simulink model "test_bu01_2018b_tuning"  (R2018b)
settings: Solver=FixedStepAuto  StartTime=0.0  StopTime=10  FixedStep=0.001  RelTol=1e-3
model workspace (MAT data in the model file):
  B1 = 0.0229925610147
  B2 = -0.371283802987
  B3 = -0.920624315565
  B4 = -0.0418343375444
  B5 = -0.493210333206
  B6 = 0
  B7 = -0.0892006103314
  B8 = -0.433620647544
  Ixx = 0.8
  Iyy = 2.075
  Izz = 1.25
  K = 0.92
  K1 = 0.96
  M1 = [1 1 -1 0.151123095698]
  M2 = [1 0 1 0.728919165533]
  M3 = [-1 0 -1 0]
  M4 = [-1 1 1 0.279370204784]
  M5 = [0 -1 0 0.953177368176]
  M6 = [0 -1 0 -1]
  M7 = [0 -1 0 0.164756597211]
  M8 = [0 -1 0 0.72330475505]
  Mass = 11.5
  b = 0
libraries: simulink x4, vrlib x4, shared6dof x1
(part 3 of 3)

== system test_bu01_2018b_tuning/Plant/bu01_model/动力系统模型/Motor4_TM_N/TM1654N /螺旋桨模型/螺旋桨气动/计算螺旋桨气动系数 ==
  In1 : Inport
  Bus Selector : BusSelector  OutputSignals=Miu,Lumda
  Mux : Mux  Inputs=6
  计算Cmx : Subsystem
  计算Cmy : Subsystem
  计算Cmz : Subsystem
  计算Ctx : Subsystem
  计算Cty : Subsystem
  计算Ctz : Subsystem
  Out1 : Outport
  wires:
  In1/1 -> Bus Selector/1
  Bus Selector/1 -> 计算Cmz/1(Miu), 计算Cmy/1(Miu), 计算Cmx/1(Miu), 计算Ctz/1(Miu), 计算Cty/1(Miu), 计算Ctx/1(Miu)  "<Miu>"
  Bus Selector/2 -> 计算Cmz/2(Lumda), 计算Cmy/2(Lumda), 计算Cmx/2(Lumda), 计算Ctz/2(Lumda), 计算Ctx/2(Lumda), 计算Cty/2(Lumda)  "<Lumda>"
  计算Ctx/1(Ctx) -> Mux/1  "Ctx"
  计算Cty/1(Cty) -> Mux/2  "Cty"
  计算Ctz/1(Ctz) -> Mux/3  "Ctz"
  计算Cmx/1(Cmx) -> Mux/4  "Cmx"
  计算Cmy/1(Cmy) -> Mux/5  "Cmy"
  计算Cmz/1(Cmz) -> Mux/6  "Cmz"
  Mux/1 -> Out1/1

== system test_bu01_2018b_tuning/Plant/bu01_model/动力系统模型/Motor5_PF_N/PF70mmDuctFanN/涵道风扇模型 /求解涵道风扇气动载荷/Fxp ==
  Vha : Inport
  Vva1 : Inport  Port=2
  Ns : Inport  Port=3
  -0.00000028262 : Gain  Gain=-0.00000028262
  -0.0038 : Gain  Gain=-0.0038
  -0.005 : Gain  Gain=-0.005
  -0.1371 : Gain  Gain=-0.1371
  0.00019569 : Gain  Gain=0.00019569
  Ns^2 : Math  Operator=square  SaturateOnIntegerOverflow=on
  Plus : Sum  Inputs=+++++
  Vha*Ns^2 : Product
  Vha*Vva1 : Product
  Vha*Vva1^2 : Product
  Vha^2 : Math  Operator=square  SaturateOnIntegerOverflow=on
  Vva1^2 : Math  Operator=square  SaturateOnIntegerOverflow=on
  Out1 : Outport
  wires:
  Vha/1 -> Vha*Vva1^2/2, -0.1371/1, Vha^2/1, Vha*Ns^2/1, Vha*Vva1/1  "Vha"
  Vva1/1 -> Vva1^2/1, Vha*Vva1/2  "Vva1"
  Vha*Vva1/1 -> -0.0038/1
  -0.0038/1 -> Plus/1
  Ns/1 -> Ns^2/1  "Ns"
  Vva1^2/1 -> Vha*Vva1^2/1
  Vha*Vva1^2/1 -> 0.00019569/1
  0.00019569/1 -> Plus/2
  -0.1371/1 -> Plus/3
  Vha^2/1 -> -0.005/1
  -0.005/1 -> Plus/4
  Ns^2/1 -> Vha*Ns^2/2
  Vha*Ns^2/1 -> -0.00000028262/1
  -0.00000028262/1 -> Plus/5
  Plus/1 -> Out1/1  "Fxp"

== system test_bu01_2018b_tuning/Plant/bu01_model/动力系统模型/Motor5_PF_N/PF70mmDuctFanN/涵道风扇模型 /求解涵道风扇气动载荷/Fzp ==
  Vha : Inport
  Vva1 : Inport  Port=2
  Ns : Inport  Port=3
  -0.3033 : Gain  Gain=-0.3033
  0.000030466 : Gain  Gain=0.000030466
  0.0019 : Gain  Gain=0.0019
  0.0043 : Gain  Gain=0.0043
  Ns^2 : Math  Operator=square  SaturateOnIntegerOverflow=on
  Plus : Sum  Inputs=++++
  Vha^2 : Math  Operator=square  SaturateOnIntegerOverflow=on
  Vva1^2 : Math  Operator=square  SaturateOnIntegerOverflow=on
  Out1 : Outport
  wires:
  Vha/1 -> Vha^2/1  "Vha"
  Vva1/1 -> -0.3033/1, Vva1^2/1  "Vva1"
  Ns/1 -> Ns^2/1  "Ns"
  -0.3033/1 -> Plus/1
  Vva1^2/1 -> 0.0019/1
  0.0019/1 -> Plus/2
  Vha^2/1 -> 0.0043/1
  0.0043/1 -> Plus/3
  Ns^2/1 -> 0.000030466/1
  0.000030466/1 -> Plus/4
  Plus/1 -> Out1/1  "Fzp"

== system test_bu01_2018b_tuning/Plant/bu01_model/动力系统模型/Motor5_PF_N/PF70mmDuctFanN/涵道风扇模型 /求解涵道风扇气动载荷/Myp ==
  Vha : Inport
  Vva : Inport  Port=2
  Ns : Inport  Port=3
  -0.000000034015 : Gain  Gain=-0.000000034015
  -0.0000031711 : Gain  Gain=-0.0000031711
  -0.0158 : Gain  Gain=-0.0158
  0.000063804 : Gain  Gain=0.000063804
  0.00011649 : Gain  Gain=0.00011649
  Ns^2 : Math  Operator=square  SaturateOnIntegerOverflow=on
  Plus : Sum  Inputs=+++++
  Vha*Ns^2 : Product
  Vha*Vva1 : Product
  Vha*Vva1^2 : Product
  Vha^2 : Math  Operator=square  SaturateOnIntegerOverflow=on
  Vva1^2 : Math  Operator=square  SaturateOnIntegerOverflow=on
  Out1 : Outport
  wires:
  Vha/1 -> Vha*Vva1^2/1, -0.0158/1, Vha^2/1, Vha*Ns^2/1, Vha*Vva1/1  "Vha"
  Vva/1 -> Vha*Vva1/2, Vva1^2/1  "Vva1"
  Ns/1 -> Ns^2/1  "Ns"
  Plus/1 -> Out1/1  "Myp"
  Vha*Vva1/1 -> 0.00011649/1
  0.00011649/1 -> Plus/1
  Vha*Vva1^2/1 -> -0.0000031711/1
  -0.0000031711/1 -> Plus/2
  Vva1^2/1 -> Vha*Vva1^2/2
  -0.0158/1 -> Plus/3
  Vha^2/1 -> 0.000063804/1
  0.000063804/1 -> Plus/4
  -0.000000034015/1 -> Plus/5
  Vha*Ns^2/1 -> -0.000000034015/1
  Ns^2/1 -> Vha*Ns^2/2

== system test_bu01_2018b_tuning/Plant/bu01_model/动力系统模型/Motor5_PF_N/PF70mmDuctFanN/涵道风扇模型 /求解涵道风扇气动载荷/Mzp ==
  Vha : Inport
  Vva1 : Inport  Port=2
  Ns : Inport  Port=3
  -0.0000028793 : Gain  Gain=-0.0000028793
  -0.0002934 : Gain  Gain=-0.0002934
  -0.00035119 : Gain  Gain=-0.00035119
  "0.0000003498 " : Gain  Gain=0.0000003498
  0.000020926 : Gain  Gain=0.000020926
  Ns^2 : Math  Operator=square  SaturateOnIntegerOverflow=on
  Plus : Sum  Inputs=+++++
  Vha^2 : Math  Operator=square  SaturateOnIntegerOverflow=on
  Vva1^2 : Math  Operator=square  SaturateOnIntegerOverflow=on
  Out1 : Outport
  wires:
  Plus/1 -> Out1/1  "Mzp"
  Vha/1 -> Vha^2/1, -0.0002934/1  "Vha"
  Vva1/1 -> Vva1^2/1, -0.00035119/1  "Vva1"
  Ns/1 -> Ns^2/1  "Ns"
  -0.00035119/1 -> Plus/1
  -0.0000028793/1 -> Plus/2
  Vva1^2/1 -> -0.0000028793/1
  -0.0002934/1 -> Plus/3
  0.000020926/1 -> Plus/4
  Vha^2/1 -> 0.000020926/1
  "0.0000003498 "/1 -> Plus/5
  Ns^2/1 -> "0.0000003498 "/1

== system test_bu01_2018b_tuning/Plant/bu01_model/动力系统模型/Motor5_PF_N/PF70mmDuctFanN/涵道风扇模型 /求解涵道风扇气动载荷/切向速度低 ==
  Ax : Inport
  Fp : Inport  Port=2
  Mp : Inport  Port=3
  Bus Creator : BusCreator  Inputs=2
  Matrix Multiply : Product
  Matrix Multiply1 : Product
  Out1 : Outport
  wires:
  Ax/1 -> Matrix Multiply1/2, Matrix Multiply/2  "Ax"
  Fp/1 -> Matrix Multiply/1  "Fp"
  Mp/1 -> Matrix Multiply1/1  "Mp"
  Bus Creator/1 -> Out1/1
  Matrix Multiply/1 -> Bus Creator/1  "Fb"
  Matrix Multiply1/1 -> Bus Creator/2  "Mb"

== system test_bu01_2018b_tuning/Plant/bu01_model/动力系统模型/Motor5_PF_N/PF70mmDuctFanN/涵道风扇模型 /求解涵道风扇气动载荷/需要坐标转换 ==
  Az : Inport
  "[Uba, Vba, Wba]" : Inport  Port=2
  Vva : Inport  Port=3
  Vha : Inport  Port=4
  Fp : Inport  Port=5
  Mp : Inport  Port=6
  Az*Vva : Product
  Az*Vva-Vb : Sum  Inputs=+-
  Bus Creator2 : BusCreator  Inputs=2
  Cross Product : vrlib/Utilities/Cross Product
      settings: SourceProductBaseCode=VR
  Divide : Product  Inputs=*/
  Fxb : DotProduct  InputSameDT=on  OutDataTypeStr=Inherit: Inherit via internal rule
  Fyb : DotProduct  InputSameDT=on  OutDataTypeStr=Inherit: Inherit via internal rule
  Fzb : DotProduct  InputSameDT=on  OutDataTypeStr=Inherit: Inherit via internal rule
  Mux : Mux  Inputs=3
  Mux1 : Mux  Inputs=3
  Mxb : DotProduct  InputSameDT=on  OutDataTypeStr=Inherit: Inherit via internal rule
  Myb : DotProduct  InputSameDT=on  OutDataTypeStr=Inherit: Inherit via internal rule
  Mzb : DotProduct  InputSameDT=on  OutDataTypeStr=Inherit: Inherit via internal rule
  Saturation : Saturate  UpperLimit=inf  LowerLimit=eps
  Out1 : Outport
  wires:
  Vva/1 -> Az*Vva/2  "Vva"
  Az/1 -> Cross Product/1, Fzb/2, Mzb/2, Az*Vva/1  "Azb"
  Az*Vva/1 -> Az*Vva-Vb/1
  "[Uba, Vba, Wba]"/1 -> Az*Vva-Vb/2  "Vb"
  Az*Vva-Vb/1 -> Divide/1
  Divide/1 -> Cross Product/2, Mxb/2, Fxb/2  "Axb"
  Cross Product/1 -> Myb/2, Fyb/2  "Ayb"
  Fp/1 -> Fzb/1, Fyb/1, Fxb/1
  Mp/1 -> Mzb/1, Myb/1, Mxb/1
  Fxb/1 -> Mux1/1  "Fxb"
  Fyb/1 -> Mux1/2  "Fyb"
  Fzb/1 -> Mux1/3  "Fzb"
  Mxb/1 -> Mux/1  "Mxb"
  Myb/1 -> Mux/2  "Myb"
  Mzb/1 -> Mux/3  "Mzb"
  Mux1/1 -> Bus Creator2/1  "Fb"
  Mux/1 -> Bus Creator2/2  "Mb"
  Bus Creator2/1 -> Out1/1
  Vha/1 -> Saturation/1  "Vha"
  Saturation/1 -> Divide/2

== system test_bu01_2018b_tuning/Plant/bu01_model/动力系统模型/Motor6_PF_N/PF70mmDuctFanN/涵道风扇模型 /求解涵道风扇气动载荷/Fxp ==
  Vha : Inport
  Vva1 : Inport  Port=2
  Ns : Inport  Port=3
  -0.00000028262 : Gain  Gain=-0.00000028262
  -0.0038 : Gain  Gain=-0.0038
  -0.005 : Gain  Gain=-0.005
  -0.1371 : Gain  Gain=-0.1371
  0.00019569 : Gain  Gain=0.00019569
  Ns^2 : Math  Operator=square  SaturateOnIntegerOverflow=on
  Plus : Sum  Inputs=+++++
  Vha*Ns^2 : Product
  Vha*Vva1 : Product
  Vha*Vva1^2 : Product
  Vha^2 : Math  Operator=square  SaturateOnIntegerOverflow=on
  Vva1^2 : Math  Operator=square  SaturateOnIntegerOverflow=on
  Out1 : Outport
  wires:
  Vha/1 -> Vha*Vva1^2/2, -0.1371/1, Vha^2/1, Vha*Ns^2/1, Vha*Vva1/1  "Vha"
  Vva1/1 -> Vva1^2/1, Vha*Vva1/2  "Vva1"
  Vha*Vva1/1 -> -0.0038/1
  -0.0038/1 -> Plus/1
  Ns/1 -> Ns^2/1  "Ns"
  Vva1^2/1 -> Vha*Vva1^2/1
  Vha*Vva1^2/1 -> 0.00019569/1
  0.00019569/1 -> Plus/2
  -0.1371/1 -> Plus/3
  Vha^2/1 -> -0.005/1
  -0.005/1 -> Plus/4
  Ns^2/1 -> Vha*Ns^2/2
  Vha*Ns^2/1 -> -0.00000028262/1
  -0.00000028262/1 -> Plus/5
  Plus/1 -> Out1/1  "Fxp"

== system test_bu01_2018b_tuning/Plant/bu01_model/动力系统模型/Motor6_PF_N/PF70mmDuctFanN/涵道风扇模型 /求解涵道风扇气动载荷/Fzp ==
  Vha : Inport
  Vva1 : Inport  Port=2
  Ns : Inport  Port=3
  -0.3033 : Gain  Gain=-0.3033
  0.000030466 : Gain  Gain=0.000030466
  0.0019 : Gain  Gain=0.0019
  0.0043 : Gain  Gain=0.0043
  Ns^2 : Math  Operator=square  SaturateOnIntegerOverflow=on
  Plus : Sum  Inputs=++++
  Vha^2 : Math  Operator=square  SaturateOnIntegerOverflow=on
  Vva1^2 : Math  Operator=square  SaturateOnIntegerOverflow=on
  Out1 : Outport
  wires:
  Vha/1 -> Vha^2/1  "Vha"
  Vva1/1 -> -0.3033/1, Vva1^2/1  "Vva1"
  Ns/1 -> Ns^2/1  "Ns"
  -0.3033/1 -> Plus/1
  Vva1^2/1 -> 0.0019/1
  0.0019/1 -> Plus/2
  Vha^2/1 -> 0.0043/1
  0.0043/1 -> Plus/3
  Ns^2/1 -> 0.000030466/1
  0.000030466/1 -> Plus/4
  Plus/1 -> Out1/1  "Fzp"

== system test_bu01_2018b_tuning/Plant/bu01_model/动力系统模型/Motor6_PF_N/PF70mmDuctFanN/涵道风扇模型 /求解涵道风扇气动载荷/Myp ==
  Vha : Inport
  Vva : Inport  Port=2
  Ns : Inport  Port=3
  -0.000000034015 : Gain  Gain=-0.000000034015
  -0.0000031711 : Gain  Gain=-0.0000031711
  -0.0158 : Gain  Gain=-0.0158
  0.000063804 : Gain  Gain=0.000063804
  0.00011649 : Gain  Gain=0.00011649
  Ns^2 : Math  Operator=square  SaturateOnIntegerOverflow=on
  Plus : Sum  Inputs=+++++
  Vha*Ns^2 : Product
  Vha*Vva1 : Product
  Vha*Vva1^2 : Product
  Vha^2 : Math  Operator=square  SaturateOnIntegerOverflow=on
  Vva1^2 : Math  Operator=square  SaturateOnIntegerOverflow=on
  Out1 : Outport
  wires:
  Vha/1 -> Vha*Vva1^2/1, -0.0158/1, Vha^2/1, Vha*Ns^2/1, Vha*Vva1/1  "Vha"
  Vva/1 -> Vha*Vva1/2, Vva1^2/1  "Vva1"
  Ns/1 -> Ns^2/1  "Ns"
  Plus/1 -> Out1/1  "Myp"
  Vha*Vva1/1 -> 0.00011649/1
  0.00011649/1 -> Plus/1
  Vha*Vva1^2/1 -> -0.0000031711/1
  -0.0000031711/1 -> Plus/2
  Vva1^2/1 -> Vha*Vva1^2/2
  -0.0158/1 -> Plus/3
  Vha^2/1 -> 0.000063804/1
  0.000063804/1 -> Plus/4
  -0.000000034015/1 -> Plus/5
  Vha*Ns^2/1 -> -0.000000034015/1
  Ns^2/1 -> Vha*Ns^2/2

== system test_bu01_2018b_tuning/Plant/bu01_model/动力系统模型/Motor6_PF_N/PF70mmDuctFanN/涵道风扇模型 /求解涵道风扇气动载荷/Mzp ==
  Vha : Inport
  Vva1 : Inport  Port=2
  Ns : Inport  Port=3
  -0.0000028793 : Gain  Gain=-0.0000028793
  -0.0002934 : Gain  Gain=-0.0002934
  -0.00035119 : Gain  Gain=-0.00035119
  "0.0000003498 " : Gain  Gain=0.0000003498
  0.000020926 : Gain  Gain=0.000020926
  Ns^2 : Math  Operator=square  SaturateOnIntegerOverflow=on
  Plus : Sum  Inputs=+++++
  Vha^2 : Math  Operator=square  SaturateOnIntegerOverflow=on
  Vva1^2 : Math  Operator=square  SaturateOnIntegerOverflow=on
  Out1 : Outport
  wires:
  Plus/1 -> Out1/1  "Mzp"
  Vha/1 -> Vha^2/1, -0.0002934/1  "Vha"
  Vva1/1 -> Vva1^2/1, -0.00035119/1  "Vva1"
  Ns/1 -> Ns^2/1  "Ns"
  -0.00035119/1 -> Plus/1
  -0.0000028793/1 -> Plus/2
  Vva1^2/1 -> -0.0000028793/1
  -0.0002934/1 -> Plus/3
  0.000020926/1 -> Plus/4
  Vha^2/1 -> 0.000020926/1
  "0.0000003498 "/1 -> Plus/5
  Ns^2/1 -> "0.0000003498 "/1

== system test_bu01_2018b_tuning/Plant/bu01_model/动力系统模型/Motor6_PF_N/PF70mmDuctFanN/涵道风扇模型 /求解涵道风扇气动载荷/切向速度低 ==
  Ax : Inport
  Fp : Inport  Port=2
  Mp : Inport  Port=3
  Bus Creator : BusCreator  Inputs=2
  Matrix Multiply : Product
  Matrix Multiply1 : Product
  Out1 : Outport
  wires:
  Ax/1 -> Matrix Multiply1/2, Matrix Multiply/2  "Ax"
  Fp/1 -> Matrix Multiply/1  "Fp"
  Mp/1 -> Matrix Multiply1/1  "Mp"
  Bus Creator/1 -> Out1/1
  Matrix Multiply/1 -> Bus Creator/1  "Fb"
  Matrix Multiply1/1 -> Bus Creator/2  "Mb"

== system test_bu01_2018b_tuning/Plant/bu01_model/动力系统模型/Motor6_PF_N/PF70mmDuctFanN/涵道风扇模型 /求解涵道风扇气动载荷/需要坐标转换 ==
  Az : Inport
  "[Uba, Vba, Wba]" : Inport  Port=2
  Vva : Inport  Port=3
  Vha : Inport  Port=4
  Fp : Inport  Port=5
  Mp : Inport  Port=6
  Az*Vva : Product
  Az*Vva-Vb : Sum  Inputs=+-
  Bus Creator2 : BusCreator  Inputs=2
  Cross Product : vrlib/Utilities/Cross Product
      settings: SourceProductBaseCode=VR
  Divide : Product  Inputs=*/
  Fxb : DotProduct  InputSameDT=on  OutDataTypeStr=Inherit: Inherit via internal rule
  Fyb : DotProduct  InputSameDT=on  OutDataTypeStr=Inherit: Inherit via internal rule
  Fzb : DotProduct  InputSameDT=on  OutDataTypeStr=Inherit: Inherit via internal rule
  Mux : Mux  Inputs=3
  Mux1 : Mux  Inputs=3
  Mxb : DotProduct  InputSameDT=on  OutDataTypeStr=Inherit: Inherit via internal rule
  Myb : DotProduct  InputSameDT=on  OutDataTypeStr=Inherit: Inherit via internal rule
  Mzb : DotProduct  InputSameDT=on  OutDataTypeStr=Inherit: Inherit via internal rule
  Saturation : Saturate  UpperLimit=inf  LowerLimit=eps
  Out1 : Outport
  wires:
  Vva/1 -> Az*Vva/2  "Vva"
  Az/1 -> Cross Product/1, Fzb/2, Mzb/2, Az*Vva/1  "Azb"
  Az*Vva/1 -> Az*Vva-Vb/1
  "[Uba, Vba, Wba]"/1 -> Az*Vva-Vb/2  "Vb"
  Az*Vva-Vb/1 -> Divide/1
  Divide/1 -> Cross Product/2, Mxb/2, Fxb/2  "Axb"
  Cross Product/1 -> Myb/2, Fyb/2  "Ayb"
  Fp/1 -> Fzb/1, Fyb/1, Fxb/1
  Mp/1 -> Mzb/1, Myb/1, Mxb/1
  Fxb/1 -> Mux1/1  "Fxb"
  Fyb/1 -> Mux1/2  "Fyb"
  Fzb/1 -> Mux1/3  "Fzb"
  Mxb/1 -> Mux/1  "Mxb"
  Myb/1 -> Mux/2  "Myb"
  Mzb/1 -> Mux/3  "Mzb"
  Mux1/1 -> Bus Creator2/1  "Fb"
  Mux/1 -> Bus Creator2/2  "Mb"
  Bus Creator2/1 -> Out1/1
  Vha/1 -> Saturation/1  "Vha"
  Saturation/1 -> Divide/2

== system test_bu01_2018b_tuning/Plant/bu01_model/动力系统模型/Motor7_PF_N/PF70mmDuctFanN/涵道风扇模型 /求解涵道风扇气动载荷/Fxp ==
  Vha : Inport
  Vva1 : Inport  Port=2
  Ns : Inport  Port=3
  -0.00000028262 : Gain  Gain=-0.00000028262
  -0.0038 : Gain  Gain=-0.0038
  -0.005 : Gain  Gain=-0.005
  -0.1371 : Gain  Gain=-0.1371
  0.00019569 : Gain  Gain=0.00019569
  Ns^2 : Math  Operator=square  SaturateOnIntegerOverflow=on
  Plus : Sum  Inputs=+++++
  Vha*Ns^2 : Product
  Vha*Vva1 : Product
  Vha*Vva1^2 : Product
  Vha^2 : Math  Operator=square  SaturateOnIntegerOverflow=on
  Vva1^2 : Math  Operator=square  SaturateOnIntegerOverflow=on
  Out1 : Outport
  wires:
  Vha/1 -> Vha*Vva1^2/2, -0.1371/1, Vha^2/1, Vha*Ns^2/1, Vha*Vva1/1  "Vha"
  Vva1/1 -> Vva1^2/1, Vha*Vva1/2  "Vva1"
  Vha*Vva1/1 -> -0.0038/1
  -0.0038/1 -> Plus/1
  Ns/1 -> Ns^2/1  "Ns"
  Vva1^2/1 -> Vha*Vva1^2/1
  Vha*Vva1^2/1 -> 0.00019569/1
  0.00019569/1 -> Plus/2
  -0.1371/1 -> Plus/3
  Vha^2/1 -> -0.005/1
  -0.005/1 -> Plus/4
  Ns^2/1 -> Vha*Ns^2/2
  Vha*Ns^2/1 -> -0.00000028262/1
  -0.00000028262/1 -> Plus/5
  Plus/1 -> Out1/1  "Fxp"

== system test_bu01_2018b_tuning/Plant/bu01_model/动力系统模型/Motor7_PF_N/PF70mmDuctFanN/涵道风扇模型 /求解涵道风扇气动载荷/Fzp ==
  Vha : Inport
  Vva1 : Inport  Port=2
  Ns : Inport  Port=3
  -0.3033 : Gain  Gain=-0.3033
  0.000030466 : Gain  Gain=0.000030466
  0.0019 : Gain  Gain=0.0019
  0.0043 : Gain  Gain=0.0043
  Ns^2 : Math  Operator=square  SaturateOnIntegerOverflow=on
  Plus : Sum  Inputs=++++
  Vha^2 : Math  Operator=square  SaturateOnIntegerOverflow=on
  Vva1^2 : Math  Operator=square  SaturateOnIntegerOverflow=on
  Out1 : Outport
  wires:
  Vha/1 -> Vha^2/1  "Vha"
  Vva1/1 -> -0.3033/1, Vva1^2/1  "Vva1"
  Ns/1 -> Ns^2/1  "Ns"
  -0.3033/1 -> Plus/1
  Vva1^2/1 -> 0.0019/1
  0.0019/1 -> Plus/2
  Vha^2/1 -> 0.0043/1
  0.0043/1 -> Plus/3
  Ns^2/1 -> 0.000030466/1
  0.000030466/1 -> Plus/4
  Plus/1 -> Out1/1  "Fzp"

== system test_bu01_2018b_tuning/Plant/bu01_model/动力系统模型/Motor7_PF_N/PF70mmDuctFanN/涵道风扇模型 /求解涵道风扇气动载荷/Myp ==
  Vha : Inport
  Vva : Inport  Port=2
  Ns : Inport  Port=3
  -0.000000034015 : Gain  Gain=-0.000000034015
  -0.0000031711 : Gain  Gain=-0.0000031711
  -0.0158 : Gain  Gain=-0.0158
  0.000063804 : Gain  Gain=0.000063804
  0.00011649 : Gain  Gain=0.00011649
  Ns^2 : Math  Operator=square  SaturateOnIntegerOverflow=on
  Plus : Sum  Inputs=+++++
  Vha*Ns^2 : Product
  Vha*Vva1 : Product
  Vha*Vva1^2 : Product
  Vha^2 : Math  Operator=square  SaturateOnIntegerOverflow=on
  Vva1^2 : Math  Operator=square  SaturateOnIntegerOverflow=on
  Out1 : Outport
  wires:
  Vha/1 -> Vha*Vva1^2/1, -0.0158/1, Vha^2/1, Vha*Ns^2/1, Vha*Vva1/1  "Vha"
  Vva/1 -> Vha*Vva1/2, Vva1^2/1  "Vva1"
  Ns/1 -> Ns^2/1  "Ns"
  Plus/1 -> Out1/1  "Myp"
  Vha*Vva1/1 -> 0.00011649/1
  0.00011649/1 -> Plus/1
  Vha*Vva1^2/1 -> -0.0000031711/1
  -0.0000031711/1 -> Plus/2
  Vva1^2/1 -> Vha*Vva1^2/2
  -0.0158/1 -> Plus/3
  Vha^2/1 -> 0.000063804/1
  0.000063804/1 -> Plus/4
  -0.000000034015/1 -> Plus/5
  Vha*Ns^2/1 -> -0.000000034015/1
  Ns^2/1 -> Vha*Ns^2/2

== system test_bu01_2018b_tuning/Plant/bu01_model/动力系统模型/Motor7_PF_N/PF70mmDuctFanN/涵道风扇模型 /求解涵道风扇气动载荷/Mzp ==
  Vha : Inport
  Vva1 : Inport  Port=2
  Ns : Inport  Port=3
  -0.0000028793 : Gain  Gain=-0.0000028793
  -0.0002934 : Gain  Gain=-0.0002934
  -0.00035119 : Gain  Gain=-0.00035119
  "0.0000003498 " : Gain  Gain=0.0000003498
  0.000020926 : Gain  Gain=0.000020926
  Ns^2 : Math  Operator=square  SaturateOnIntegerOverflow=on
  Plus : Sum  Inputs=+++++
  Vha^2 : Math  Operator=square  SaturateOnIntegerOverflow=on
  Vva1^2 : Math  Operator=square  SaturateOnIntegerOverflow=on
  Out1 : Outport
  wires:
  Plus/1 -> Out1/1  "Mzp"
  Vha/1 -> Vha^2/1, -0.0002934/1  "Vha"
  Vva1/1 -> Vva1^2/1, -0.00035119/1  "Vva1"
  Ns/1 -> Ns^2/1  "Ns"
  -0.00035119/1 -> Plus/1
  -0.0000028793/1 -> Plus/2
  Vva1^2/1 -> -0.0000028793/1
  -0.0002934/1 -> Plus/3
  0.000020926/1 -> Plus/4
  Vha^2/1 -> 0.000020926/1
  "0.0000003498 "/1 -> Plus/5
  Ns^2/1 -> "0.0000003498 "/1

== system test_bu01_2018b_tuning/Plant/bu01_model/动力系统模型/Motor7_PF_N/PF70mmDuctFanN/涵道风扇模型 /求解涵道风扇气动载荷/切向速度低 ==
  Ax : Inport
  Fp : Inport  Port=2
  Mp : Inport  Port=3
  Bus Creator : BusCreator  Inputs=2
  Matrix Multiply : Product
  Matrix Multiply1 : Product
  Out1 : Outport
  wires:
  Ax/1 -> Matrix Multiply1/2, Matrix Multiply/2  "Ax"
  Fp/1 -> Matrix Multiply/1  "Fp"
  Mp/1 -> Matrix Multiply1/1  "Mp"
  Bus Creator/1 -> Out1/1
  Matrix Multiply/1 -> Bus Creator/1  "Fb"
  Matrix Multiply1/1 -> Bus Creator/2  "Mb"

== system test_bu01_2018b_tuning/Plant/bu01_model/动力系统模型/Motor7_PF_N/PF70mmDuctFanN/涵道风扇模型 /求解涵道风扇气动载荷/需要坐标转换 ==
  Az : Inport
  "[Uba, Vba, Wba]" : Inport  Port=2
  Vva : Inport  Port=3
  Vha : Inport  Port=4
  Fp : Inport  Port=5
  Mp : Inport  Port=6
  Az*Vva : Product
  Az*Vva-Vb : Sum  Inputs=+-
  Bus Creator2 : BusCreator  Inputs=2
  Cross Product : vrlib/Utilities/Cross Product
      settings: SourceProductBaseCode=VR
  Divide : Product  Inputs=*/
  Fxb : DotProduct  InputSameDT=on  OutDataTypeStr=Inherit: Inherit via internal rule
  Fyb : DotProduct  InputSameDT=on  OutDataTypeStr=Inherit: Inherit via internal rule
  Fzb : DotProduct  InputSameDT=on  OutDataTypeStr=Inherit: Inherit via internal rule
  Mux : Mux  Inputs=3
  Mux1 : Mux  Inputs=3
  Mxb : DotProduct  InputSameDT=on  OutDataTypeStr=Inherit: Inherit via internal rule
  Myb : DotProduct  InputSameDT=on  OutDataTypeStr=Inherit: Inherit via internal rule
  Mzb : DotProduct  InputSameDT=on  OutDataTypeStr=Inherit: Inherit via internal rule
  Saturation : Saturate  UpperLimit=inf  LowerLimit=eps
  Out1 : Outport
  wires:
  Vva/1 -> Az*Vva/2  "Vva"
  Az/1 -> Cross Product/1, Fzb/2, Mzb/2, Az*Vva/1  "Azb"
  Az*Vva/1 -> Az*Vva-Vb/1
  "[Uba, Vba, Wba]"/1 -> Az*Vva-Vb/2  "Vb"
  Az*Vva-Vb/1 -> Divide/1
  Divide/1 -> Cross Product/2, Mxb/2, Fxb/2  "Axb"
  Cross Product/1 -> Myb/2, Fyb/2  "Ayb"
  Fp/1 -> Fzb/1, Fyb/1, Fxb/1
  Mp/1 -> Mzb/1, Myb/1, Mxb/1
  Fxb/1 -> Mux1/1  "Fxb"
  Fyb/1 -> Mux1/2  "Fyb"
  Fzb/1 -> Mux1/3  "Fzb"
  Mxb/1 -> Mux/1  "Mxb"
  Myb/1 -> Mux/2  "Myb"
  Mzb/1 -> Mux/3  "Mzb"
  Mux1/1 -> Bus Creator2/1  "Fb"
  Mux/1 -> Bus Creator2/2  "Mb"
  Bus Creator2/1 -> Out1/1
  Vha/1 -> Saturation/1  "Vha"
  Saturation/1 -> Divide/2

== system test_bu01_2018b_tuning/Plant/bu01_model/动力系统模型/Motor8_PF_N/PF70mmDuctFanN/涵道风扇模型 /求解涵道风扇气动载荷/Fxp ==
  Vha : Inport
  Vva1 : Inport  Port=2
  Ns : Inport  Port=3
  -0.00000028262 : Gain  Gain=-0.00000028262
  -0.0038 : Gain  Gain=-0.0038
  -0.005 : Gain  Gain=-0.005
  -0.1371 : Gain  Gain=-0.1371
  0.00019569 : Gain  Gain=0.00019569
  Ns^2 : Math  Operator=square  SaturateOnIntegerOverflow=on
  Plus : Sum  Inputs=+++++
  Vha*Ns^2 : Product
  Vha*Vva1 : Product
  Vha*Vva1^2 : Product
  Vha^2 : Math  Operator=square  SaturateOnIntegerOverflow=on
  Vva1^2 : Math  Operator=square  SaturateOnIntegerOverflow=on
  Out1 : Outport
  wires:
  Plus/1 -> Out1/1  "Fxp"
  -0.00000028262/1 -> Plus/5
  Vha*Ns^2/1 -> -0.00000028262/1
  Ns^2/1 -> Vha*Ns^2/2
  -0.005/1 -> Plus/4
  Vha^2/1 -> -0.005/1
  -0.1371/1 -> Plus/3
  0.00019569/1 -> Plus/2
  Vha*Vva1^2/1 -> 0.00019569/1
  Vva1^2/1 -> Vha*Vva1^2/1
  Ns/1 -> Ns^2/1  "Ns"
  -0.0038/1 -> Plus/1
  Vha*Vva1/1 -> -0.0038/1
  Vva1/1 -> Vha*Vva1/2, Vva1^2/1  "Vva1"
  Vha/1 -> Vha*Vva1/1, Vha*Ns^2/1, Vha^2/1, -0.1371/1, Vha*Vva1^2/2  "Vha"

== system test_bu01_2018b_tuning/Plant/bu01_model/动力系统模型/Motor8_PF_N/PF70mmDuctFanN/涵道风扇模型 /求解涵道风扇气动载荷/Fzp ==
  Vha : Inport
  Vva1 : Inport  Port=2
  Ns : Inport  Port=3
  -0.3033 : Gain  Gain=-0.3033
  0.000030466 : Gain  Gain=0.000030466
  0.0019 : Gain  Gain=0.0019
  0.0043 : Gain  Gain=0.0043
  Ns^2 : Math  Operator=square  SaturateOnIntegerOverflow=on
  Plus : Sum  Inputs=++++
  Vha^2 : Math  Operator=square  SaturateOnIntegerOverflow=on
  Vva1^2 : Math  Operator=square  SaturateOnIntegerOverflow=on
  Out1 : Outport
  wires:
  Plus/1 -> Out1/1  "Fzp"
  0.000030466/1 -> Plus/4
  Ns^2/1 -> 0.000030466/1
  0.0043/1 -> Plus/3
  Vha^2/1 -> 0.0043/1
  0.0019/1 -> Plus/2
  Vva1^2/1 -> 0.0019/1
  -0.3033/1 -> Plus/1
  Ns/1 -> Ns^2/1  "Ns"
  Vva1/1 -> Vva1^2/1, -0.3033/1  "Vva1"
  Vha/1 -> Vha^2/1  "Vha"

== system test_bu01_2018b_tuning/Plant/bu01_model/动力系统模型/Motor8_PF_N/PF70mmDuctFanN/涵道风扇模型 /求解涵道风扇气动载荷/Myp ==
  Vha : Inport
  Vva : Inport  Port=2
  Ns : Inport  Port=3
  -0.000000034015 : Gain  Gain=-0.000000034015
  -0.0000031711 : Gain  Gain=-0.0000031711
  -0.0158 : Gain  Gain=-0.0158
  0.000063804 : Gain  Gain=0.000063804
  0.00011649 : Gain  Gain=0.00011649
  Ns^2 : Math  Operator=square  SaturateOnIntegerOverflow=on
  Plus : Sum  Inputs=+++++
  Vha*Ns^2 : Product
  Vha*Vva1 : Product
  Vha*Vva1^2 : Product
  Vha^2 : Math  Operator=square  SaturateOnIntegerOverflow=on
  Vva1^2 : Math  Operator=square  SaturateOnIntegerOverflow=on
  Out1 : Outport
  wires:
  Ns^2/1 -> Vha*Ns^2/2
  Vha*Ns^2/1 -> -0.000000034015/1
  -0.000000034015/1 -> Plus/5
  0.000063804/1 -> Plus/4
  Vha^2/1 -> 0.000063804/1
  -0.0158/1 -> Plus/3
  Vva1^2/1 -> Vha*Vva1^2/2
  -0.0000031711/1 -> Plus/2
  Vha*Vva1^2/1 -> -0.0000031711/1
  0.00011649/1 -> Plus/1
  Vha*Vva1/1 -> 0.00011649/1
  Plus/1 -> Out1/1  "Myp"
  Ns/1 -> Ns^2/1  "Ns"
  Vva/1 -> Vva1^2/1, Vha*Vva1/2  "Vva1"
  Vha/1 -> Vha*Vva1/1, Vha*Ns^2/1, Vha^2/1, -0.0158/1, Vha*Vva1^2/1  "Vha"

== system test_bu01_2018b_tuning/Plant/bu01_model/动力系统模型/Motor8_PF_N/PF70mmDuctFanN/涵道风扇模型 /求解涵道风扇气动载荷/Mzp ==
  Vha : Inport
  Vva1 : Inport  Port=2
  Ns : Inport  Port=3
  -0.0000028793 : Gain  Gain=-0.0000028793
  -0.0002934 : Gain  Gain=-0.0002934
  -0.00035119 : Gain  Gain=-0.00035119
  "0.0000003498 " : Gain  Gain=0.0000003498
  0.000020926 : Gain  Gain=0.000020926
  Ns^2 : Math  Operator=square  SaturateOnIntegerOverflow=on
  Plus : Sum  Inputs=+++++
  Vha^2 : Math  Operator=square  SaturateOnIntegerOverflow=on
  Vva1^2 : Math  Operator=square  SaturateOnIntegerOverflow=on
  Out1 : Outport
  wires:
  Ns^2/1 -> "0.0000003498 "/1
  "0.0000003498 "/1 -> Plus/5
  Vha^2/1 -> 0.000020926/1
  0.000020926/1 -> Plus/4
  -0.0002934/1 -> Plus/3
  Vva1^2/1 -> -0.0000028793/1
  -0.0000028793/1 -> Plus/2
  -0.00035119/1 -> Plus/1
  Ns/1 -> Ns^2/1  "Ns"
  Vva1/1 -> -0.00035119/1, Vva1^2/1  "Vva1"
  Vha/1 -> -0.0002934/1, Vha^2/1  "Vha"
  Plus/1 -> Out1/1  "Mzp"

== system test_bu01_2018b_tuning/Plant/bu01_model/动力系统模型/Motor8_PF_N/PF70mmDuctFanN/涵道风扇模型 /求解涵道风扇气动载荷/切向速度低 ==
  Ax : Inport
  Fp : Inport  Port=2
  Mp : Inport  Port=3
  Bus Creator : BusCreator  Inputs=2
  Matrix Multiply : Product
  Matrix Multiply1 : Product
  Out1 : Outport
  wires:
  Matrix Multiply1/1 -> Bus Creator/2  "Mb"
  Matrix Multiply/1 -> Bus Creator/1  "Fb"
  Bus Creator/1 -> Out1/1
  Mp/1 -> Matrix Multiply1/1  "Mp"
  Fp/1 -> Matrix Multiply/1  "Fp"
  Ax/1 -> Matrix Multiply/2, Matrix Multiply1/2  "Ax"

== system test_bu01_2018b_tuning/Plant/bu01_model/动力系统模型/Motor8_PF_N/PF70mmDuctFanN/涵道风扇模型 /求解涵道风扇气动载荷/需要坐标转换 ==
  Az : Inport
  "[Uba, Vba, Wba]" : Inport  Port=2
  Vva : Inport  Port=3
  Vha : Inport  Port=4
  Fp : Inport  Port=5
  Mp : Inport  Port=6
  Az*Vva : Product
  Az*Vva-Vb : Sum  Inputs=+-
  Bus Creator2 : BusCreator  Inputs=2
  Cross Product : vrlib/Utilities/Cross Product
      settings: SourceProductBaseCode=VR
  Divide : Product  Inputs=*/
  Fxb : DotProduct  InputSameDT=on  OutDataTypeStr=Inherit: Inherit via internal rule
  Fyb : DotProduct  InputSameDT=on  OutDataTypeStr=Inherit: Inherit via internal rule
  Fzb : DotProduct  InputSameDT=on  OutDataTypeStr=Inherit: Inherit via internal rule
  Mux : Mux  Inputs=3
  Mux1 : Mux  Inputs=3
  Mxb : DotProduct  InputSameDT=on  OutDataTypeStr=Inherit: Inherit via internal rule
  Myb : DotProduct  InputSameDT=on  OutDataTypeStr=Inherit: Inherit via internal rule
  Mzb : DotProduct  InputSameDT=on  OutDataTypeStr=Inherit: Inherit via internal rule
  Saturation : Saturate  UpperLimit=inf  LowerLimit=eps
  Out1 : Outport
  wires:
  Bus Creator2/1 -> Out1/1
  Mux/1 -> Bus Creator2/2  "Mb"
  Mux1/1 -> Bus Creator2/1  "Fb"
  Mzb/1 -> Mux/3  "Mzb"
  Myb/1 -> Mux/2  "Myb"
  Mxb/1 -> Mux/1  "Mxb"
  Fzb/1 -> Mux1/3  "Fzb"
  Fyb/1 -> Mux1/2  "Fyb"
  Fxb/1 -> Mux1/1  "Fxb"
  Mp/1 -> Mxb/1, Myb/1, Mzb/1
  Fp/1 -> Fxb/1, Fyb/1, Fzb/1
  Cross Product/1 -> Fyb/2, Myb/2  "Ayb"
  Divide/1 -> Fxb/2, Mxb/2, Cross Product/2  "Axb"
  Az*Vva-Vb/1 -> Divide/1
  "[Uba, Vba, Wba]"/1 -> Az*Vva-Vb/2  "Vb"
  Az*Vva/1 -> Az*Vva-Vb/1
  Az/1 -> Az*Vva/1, Mzb/2, Fzb/2, Cross Product/1  "Azb"
  Vva/1 -> Az*Vva/2  "Vva"
  Vha/1 -> Saturation/1  "Vha"
  Saturation/1 -> Divide/2

== system test_bu01_2018b_tuning/Plant/bu01_model/动力系统模型/Motor1_TM_P/TM1654P /螺旋桨模型/螺旋桨气动/计算螺旋桨气动系数/计算Cmx ==
  Miu : Inport
  Lumda : Inport  Port=2
  Add : Sum  Inputs=++--
  Constant : Constant  Value=0.0101
  Gain : Gain  Gain=0.0041
  Gain1 : Gain  Gain=0.009
  Gain2 : Gain  Gain=0.0032
  Multiply : Product
  Square : Math  Operator=square  SaturateOnIntegerOverflow=on
  Cmx : Outport
  wires:
  Multiply/1 -> Cmx/1  "Cmx"
  Lumda/1 -> Square/1, Gain1/1
  Gain2/1 -> Add/4
  Square/1 -> Gain2/1
  Gain/1 -> Add/2
  Constant/1 -> Add/1
  Miu/1 -> Gain/1, Multiply/1
  Gain1/1 -> Add/3
  Add/1 -> Multiply/2

== system test_bu01_2018b_tuning/Plant/bu01_model/动力系统模型/Motor1_TM_P/TM1654P /螺旋桨模型/螺旋桨气动/计算螺旋桨气动系数/计算Cmy ==
  Miu : Inport
  Lumda : Inport  Port=2
  Add1 : Sum  Inputs=++++-
  Constant : Constant  Value=3
  Constant1 : Constant  Value=-0.015
  Gain1 : Gain  Gain=0.0115
  Gain2 : Gain  Gain=0.1908
  Gain3 : Gain  Gain=0.0146
  Gain4 : Gain  Gain=0.0484
  Multiply1 : Product
  Power : Math  Operator=pow  SaturateOnIntegerOverflow=on
  Square2 : Math  Operator=square  SaturateOnIntegerOverflow=on
  Cmy : Outport
  wires:
  Gain2/1 -> Add1/5
  Power/1 -> Gain2/1
  Constant/1 -> Power/2
  Miu/1 -> Multiply1/1, Gain1/1
  Constant1/1 -> Add1/1
  Add1/1 -> Multiply1/2
  Gain4/1 -> Add1/4
  Square2/1 -> Gain4/1
  Lumda/1 -> Square2/1, Power/1, Gain3/1
  Gain3/1 -> Add1/3
  Multiply1/1 -> Cmy/1  "Cmy"
  Gain1/1 -> Add1/2

== system test_bu01_2018b_tuning/Plant/bu01_model/动力系统模型/Motor1_TM_P/TM1654P /螺旋桨模型/螺旋桨气动/计算螺旋桨气动系数/计算Cmz ==
  Miu : Inport
  Lumda : Inport  Port=2
  Add2 : Sum  Inputs=+-+--
  Add3 : Sum  Inputs=+-++
  Constant3 : Constant  Value=0.0036
  Constant4 : Constant  Value=0.0023
  Gain10 : Gain  Gain=0.0105
  Gain11 : Gain  Gain=0.0078
  Gain6 : Gain  Gain=0.0006554
  Gain7 : Gain  Gain=0.00080732
  Gain8 : Gain  Gain=0.006
  Gain9 : Gain  Gain=0.0043
  Lumda1 : InportShadow  Port=2
  Multiply2 : Product
  Square3 : Math  Operator=square  SaturateOnIntegerOverflow=on
  Square4 : Math  Operator=square  SaturateOnIntegerOverflow=on
  Square5 : Math  Operator=square  SaturateOnIntegerOverflow=on
  Cmz : Outport
  wires:
  Lumda1/1 -> Multiply2/1
  Gain10/1 -> Add2/4
  Square3/1 -> Gain7/1
  Gain8/1 -> Add2/1
  Gain11/1 -> Add2/5
  Square5/1 -> Gain11/1
  Gain9/1 -> Add2/2
  Constant4/1 -> Add2/3
  Square4/1 -> Gain9/1
  Add2/1 -> Multiply2/2
  Constant3/1 -> Add3/1
  Lumda/1 -> Gain10/1, Square5/1
  Miu/1 -> Gain6/1, Square3/1, Square4/1, Gain8/1
  Add3/1 -> Cmz/1  "Cmz"
  Multiply2/1 -> Add3/4
  Gain6/1 -> Add3/2
  Gain7/1 -> Add3/3

== system test_bu01_2018b_tuning/Plant/bu01_model/动力系统模型/Motor1_TM_P/TM1654P /螺旋桨模型/螺旋桨气动/计算螺旋桨气动系数/计算Ctx ==
  Miu : Inport
  Lumda : Inport  Port=2
  Add : Sum  Inputs=++-+
  Constant : Constant  Value=-0.0074
  Gain : Gain  Gain=0.00051704
  Gain1 : Gain  Gain=0.0073
  Gain2 : Gain  Gain=0.018
  Multiply : Product
  Square : Math  Operator=square  SaturateOnIntegerOverflow=on
  Ctx : Outport
  wires:
  Add/1 -> Multiply/2
  Gain1/1 -> Add/3
  Miu/1 -> Multiply/1, Gain/1
  Constant/1 -> Add/1
  Gain/1 -> Add/2
  Square/1 -> Gain2/1
  Gain2/1 -> Add/4
  Lumda/1 -> Square/1, Gain1/1
  Multiply/1 -> Ctx/1  "Ctx"

== system test_bu01_2018b_tuning/Plant/bu01_model/动力系统模型/Motor1_TM_P/TM1654P /螺旋桨模型/螺旋桨气动/计算螺旋桨气动系数/计算Cty ==
  Miu : Inport
  Lumda : Inport  Port=2
  Add1 : Sum  Inputs=+++-
  Constant : Constant  Value=3
  Constant1 : Constant  Value=-0.002  OutDataTypeStr=double
  Gain3 : Gain  Gain=0.0103
  Gain4 : Gain  Gain=0.0168
  Gain5 : Gain  Gain=0.0897
  Multiply1 : Product
  Power : Math  Operator=pow  SaturateOnIntegerOverflow=on
  Square2 : Math  Operator=square  SaturateOnIntegerOverflow=on
  Cty : Outport
  wires:
  Gain5/1 -> Add1/4
  Multiply1/1 -> Cty/1  "Cty"
  Gain3/1 -> Add1/2
  Lumda/1 -> Power/1, Square2/1, Gain3/1
  Square2/1 -> Gain4/1
  Constant/1 -> Power/2
  Gain4/1 -> Add1/3
  Add1/1 -> Multiply1/2
  Constant1/1 -> Add1/1
  Power/1 -> Gain5/1
  Miu/1 -> Multiply1/1

== system test_bu01_2018b_tuning/Plant/bu01_model/动力系统模型/Motor1_TM_P/TM1654P /螺旋桨模型/螺旋桨气动/计算螺旋桨气动系数/计算Ctz ==
  Miu : Inport
  Lumda : Inport  Port=2
  Add2 : Sum  Inputs=++-+-
  Add3 : Sum  Inputs=++-+
  Constant3 : Constant  Value=0.0651
  Constant4 : Constant  Value=0.0845
  Gain10 : Gain  Gain=0.0583
  Gain11 : Gain  Gain=0.3529
  Gain6 : Gain  Gain=0.0579
  Gain7 : Gain  Gain=0.0066
  Gain8 : Gain  Gain=-0.2325
  Gain9 : Gain  Gain=0.1346
  Lumda1 : InportShadow  Port=2
  Multiply2 : Product
  Square3 : Math  Operator=square  SaturateOnIntegerOverflow=on
  Square4 : Math  Operator=square  SaturateOnIntegerOverflow=on
  Square5 : Math  Operator=square  SaturateOnIntegerOverflow=on
  Ctz : Outport
  wires:
  Gain7/1 -> Add3/3
  Gain6/1 -> Add3/2
  Multiply2/1 -> Add3/4
  Add3/1 -> Ctz/1  "Ctz"
  Miu/1 -> Square4/1, Gain6/1, Square3/1, Gain8/1
  Lumda/1 -> Square5/1, Gain10/1
  Constant3/1 -> Add3/1
  Add2/1 -> Multiply2/2
  Square4/1 -> Gain9/1
  Constant4/1 -> Add2/3
  Gain9/1 -> Add2/2
  Square5/1 -> Gain11/1
  Gain11/1 -> Add2/5
  Gain8/1 -> Add2/1
  Square3/1 -> Gain7/1
  Gain10/1 -> Add2/4
  Lumda1/1 -> Multiply2/1

== system test_bu01_2018b_tuning/Plant/bu01_model/动力系统模型/Motor2_TM_N/TM1654N /螺旋桨模型/螺旋桨气动/计算螺旋桨气动系数/计算Cmx ==
  Miu : Inport
  Lumda : Inport  Port=2
  Add : Sum  Inputs=++--
  Constant : Constant  Value=0.0101
  Gain : Gain  Gain=0.0041
  Gain1 : Gain  Gain=0.009
  Gain2 : Gain  Gain=0.0032
  Multiply : Product
  Square : Math  Operator=square  SaturateOnIntegerOverflow=on
  Cmx : Outport
  wires:
  Multiply/1 -> Cmx/1  "Cmx"
  Lumda/1 -> Square/1, Gain1/1
  Gain2/1 -> Add/4
  Square/1 -> Gain2/1
  Gain/1 -> Add/2
  Constant/1 -> Add/1
  Miu/1 -> Multiply/1, Gain/1
  Gain1/1 -> Add/3
  Add/1 -> Multiply/2

== system test_bu01_2018b_tuning/Plant/bu01_model/动力系统模型/Motor2_TM_N/TM1654N /螺旋桨模型/螺旋桨气动/计算螺旋桨气动系数/计算Cmy ==
  Miu : Inport
  Lumda : Inport  Port=2
  Add1 : Sum  Inputs=++--
  Constant1 : Constant  Value=0.0101
  Gain1 : Gain  Gain=0.0041
  Gain3 : Gain  Gain=0.009
  Gain4 : Gain  Gain=0.0032
  Multiply1 : Product
  Square2 : Math  Operator=square  SaturateOnIntegerOverflow=on
  Cmy : Outport
  wires:
  Miu/1 -> Multiply1/1, Gain1/1
  Constant1/1 -> Add1/1
  Add1/1 -> Multiply1/2
  Gain4/1 -> Add1/4
  Square2/1 -> Gain4/1
  Lumda/1 -> Square2/1, Gain3/1
  Gain3/1 -> Add1/3
  Multiply1/1 -> Cmy/1  "Cmy"
  Gain1/1 -> Add1/2

== system test_bu01_2018b_tuning/Plant/bu01_model/动力系统模型/Motor2_TM_N/TM1654N /螺旋桨模型/螺旋桨气动/计算螺旋桨气动系数/计算Cmz ==
  Miu : Inport
  Lumda : Inport  Port=2
  Add2 : Sum  Inputs=+-+--
  Add3 : Sum  Inputs=+-++
  Constant3 : Constant  Value=0.0036
  Constant4 : Constant  Value=0.0023
  Gain10 : Gain  Gain=0.0105
  Gain11 : Gain  Gain=0.0078
  Gain6 : Gain  Gain=0.0006554
  Gain7 : Gain  Gain=0.00080732
  Gain8 : Gain  Gain=0.006
  Gain9 : Gain  Gain=0.0043
  Lumda1 : InportShadow  Port=2
  Multiply2 : Product
  Square3 : Math  Operator=square  SaturateOnIntegerOverflow=on
  Square4 : Math  Operator=square  SaturateOnIntegerOverflow=on
  Square5 : Math  Operator=square  SaturateOnIntegerOverflow=on
  Cmz : Outport
  wires:
  Lumda1/1 -> Multiply2/1
  Gain10/1 -> Add2/4
  Square3/1 -> Gain7/1
  Gain8/1 -> Add2/1
  Gain11/1 -> Add2/5
  Square5/1 -> Gain11/1
  Gain9/1 -> Add2/2
  Constant4/1 -> Add2/3
  Square4/1 -> Gain9/1
  Add2/1 -> Multiply2/2
  Constant3/1 -> Add3/1
  Lumda/1 -> Gain10/1, Square5/1
  Miu/1 -> Gain6/1, Square3/1, Square4/1, Gain8/1
  Add3/1 -> Cmz/1  "Cmz"
  Multiply2/1 -> Add3/4
  Gain6/1 -> Add3/2
  Gain7/1 -> Add3/3

== system test_bu01_2018b_tuning/Plant/bu01_model/动力系统模型/Motor2_TM_N/TM1654N /螺旋桨模型/螺旋桨气动/计算螺旋桨气动系数/计算Ctx ==
  Miu : Inport
  Lumda : Inport  Port=2
  Add : Sum  Inputs=++-+
  Constant : Constant  Value=-0.0074
  Gain : Gain  Gain=0.00051704
  Gain1 : Gain  Gain=0.0073
  Gain2 : Gain  Gain=0.018
  Multiply : Product
  Square : Math  Operator=square  SaturateOnIntegerOverflow=on
  Ctx : Outport
  wires:
  Add/1 -> Multiply/2
  Gain1/1 -> Add/3
  Miu/1 -> Multiply/1, Gain/1
  Constant/1 -> Add/1
  Gain/1 -> Add/2
  Square/1 -> Gain2/1
  Gain2/1 -> Add/4
  Lumda/1 -> Square/1, Gain1/1
  Multiply/1 -> Ctx/1  "Ctx"

== system test_bu01_2018b_tuning/Plant/bu01_model/动力系统模型/Motor2_TM_N/TM1654N /螺旋桨模型/螺旋桨气动/计算螺旋桨气动系数/计算Cty ==
  Miu : Inport
  Lumda : Inport  Port=2
  Add1 : Sum  Inputs=+++-
  Constant : Constant  Value=3
  Constant1 : Constant  Value=-0.002  OutDataTypeStr=double
  Gain3 : Gain  Gain=0.0103
  Gain4 : Gain  Gain=0.0168
  Gain5 : Gain  Gain=0.0897
  Multiply1 : Product
  Power : Math  Operator=pow  SaturateOnIntegerOverflow=on
  Square2 : Math  Operator=square  SaturateOnIntegerOverflow=on
  Cty : Outport
  wires:
  Gain5/1 -> Add1/4
  Multiply1/1 -> Cty/1  "Cty"
  Gain3/1 -> Add1/2
  Lumda/1 -> Power/1, Square2/1, Gain3/1
  Square2/1 -> Gain4/1
  Constant/1 -> Power/2
  Gain4/1 -> Add1/3
  Add1/1 -> Multiply1/2
  Constant1/1 -> Add1/1
  Power/1 -> Gain5/1
  Miu/1 -> Multiply1/1

== system test_bu01_2018b_tuning/Plant/bu01_model/动力系统模型/Motor2_TM_N/TM1654N /螺旋桨模型/螺旋桨气动/计算螺旋桨气动系数/计算Ctz ==
  Miu : Inport
  Lumda : Inport  Port=2
  Add2 : Sum  Inputs=++-+-
  Add3 : Sum  Inputs=++-+
  Constant3 : Constant  Value=0.0651
  Constant4 : Constant  Value=0.0845
  Gain10 : Gain  Gain=0.0583
  Gain11 : Gain  Gain=0.3529
  Gain6 : Gain  Gain=0.0579
  Gain7 : Gain  Gain=0.0066
  Gain8 : Gain  Gain=-0.2325
  Gain9 : Gain  Gain=0.1346
  Lumda1 : InportShadow  Port=2
  Multiply2 : Product
  Square3 : Math  Operator=square  SaturateOnIntegerOverflow=on
  Square4 : Math  Operator=square  SaturateOnIntegerOverflow=on
  Square5 : Math  Operator=square  SaturateOnIntegerOverflow=on
  Ctz : Outport
  wires:
  Gain7/1 -> Add3/3
  Gain6/1 -> Add3/2
  Multiply2/1 -> Add3/4
  Add3/1 -> Ctz/1  "Ctz"
  Miu/1 -> Gain8/1, Square4/1, Square3/1, Gain6/1
  Lumda/1 -> Square5/1, Gain10/1
  Constant3/1 -> Add3/1
  Add2/1 -> Multiply2/2
  Square4/1 -> Gain9/1
  Constant4/1 -> Add2/3
  Gain9/1 -> Add2/2
  Square5/1 -> Gain11/1
  Gain11/1 -> Add2/5
  Gain8/1 -> Add2/1
  Square3/1 -> Gain7/1
  Gain10/1 -> Add2/4
  Lumda1/1 -> Multiply2/1

== system test_bu01_2018b_tuning/Plant/bu01_model/动力系统模型/Motor3_TM_P/TM1654P /螺旋桨模型/螺旋桨气动/计算螺旋桨气动系数/计算Cmx ==
  Miu : Inport
  Lumda : Inport  Port=2
  Add : Sum  Inputs=++--
  Constant : Constant  Value=0.0101
  Gain : Gain  Gain=0.0041
  Gain1 : Gain  Gain=0.009
  Gain2 : Gain  Gain=0.0032
  Multiply : Product
  Square : Math  Operator=square  SaturateOnIntegerOverflow=on
  Cmx : Outport
  wires:
  Multiply/1 -> Cmx/1  "Cmx"
  Lumda/1 -> Square/1, Gain1/1
  Gain2/1 -> Add/4
  Square/1 -> Gain2/1
  Gain/1 -> Add/2
  Constant/1 -> Add/1
  Miu/1 -> Gain/1, Multiply/1
  Gain1/1 -> Add/3
  Add/1 -> Multiply/2

== system test_bu01_2018b_tuning/Plant/bu01_model/动力系统模型/Motor3_TM_P/TM1654P /螺旋桨模型/螺旋桨气动/计算螺旋桨气动系数/计算Cmy ==
  Miu : Inport
  Lumda : Inport  Port=2
  Add1 : Sum  Inputs=++++-
  Constant : Constant  Value=3
  Constant1 : Constant  Value=-0.015
  Gain1 : Gain  Gain=0.0115
  Gain2 : Gain  Gain=0.1908
  Gain3 : Gain  Gain=0.0146
  Gain4 : Gain  Gain=0.0484
  Multiply1 : Product
  Power : Math  Operator=pow  SaturateOnIntegerOverflow=on
  Square2 : Math  Operator=square  SaturateOnIntegerOverflow=on
  Cmy : Outport
  wires:
  Gain2/1 -> Add1/5
  Power/1 -> Gain2/1
  Constant/1 -> Power/2
  Miu/1 -> Multiply1/1, Gain1/1
  Constant1/1 -> Add1/1
  Add1/1 -> Multiply1/2
  Gain4/1 -> Add1/4
  Square2/1 -> Gain4/1
  Lumda/1 -> Square2/1, Power/1, Gain3/1
  Gain3/1 -> Add1/3
  Multiply1/1 -> Cmy/1  "Cmy"
  Gain1/1 -> Add1/2

== system test_bu01_2018b_tuning/Plant/bu01_model/动力系统模型/Motor3_TM_P/TM1654P /螺旋桨模型/螺旋桨气动/计算螺旋桨气动系数/计算Cmz ==
  Miu : Inport
  Lumda : Inport  Port=2
  Add2 : Sum  Inputs=+-+--
  Add3 : Sum  Inputs=+-++
  Constant3 : Constant  Value=0.0036
  Constant4 : Constant  Value=0.0023
  Gain10 : Gain  Gain=0.0105
  Gain11 : Gain  Gain=0.0078
  Gain6 : Gain  Gain=0.0006554
  Gain7 : Gain  Gain=0.00080732
  Gain8 : Gain  Gain=0.006
  Gain9 : Gain  Gain=0.0043
  Lumda1 : InportShadow  Port=2
  Multiply2 : Product
  Square3 : Math  Operator=square  SaturateOnIntegerOverflow=on
  Square4 : Math  Operator=square  SaturateOnIntegerOverflow=on
  Square5 : Math  Operator=square  SaturateOnIntegerOverflow=on
  Cmz : Outport
  wires:
  Lumda1/1 -> Multiply2/1
  Gain10/1 -> Add2/4
  Square3/1 -> Gain7/1
  Gain8/1 -> Add2/1
  Gain11/1 -> Add2/5
  Square5/1 -> Gain11/1
  Gain9/1 -> Add2/2
  Constant4/1 -> Add2/3
  Square4/1 -> Gain9/1
  Add2/1 -> Multiply2/2
  Constant3/1 -> Add3/1
  Lumda/1 -> Gain10/1, Square5/1
  Miu/1 -> Gain6/1, Square3/1, Square4/1, Gain8/1
  Add3/1 -> Cmz/1  "Cmz"
  Multiply2/1 -> Add3/4
  Gain6/1 -> Add3/2
  Gain7/1 -> Add3/3

== system test_bu01_2018b_tuning/Plant/bu01_model/动力系统模型/Motor3_TM_P/TM1654P /螺旋桨模型/螺旋桨气动/计算螺旋桨气动系数/计算Ctx ==
  Miu : Inport
  Lumda : Inport  Port=2
  Add : Sum  Inputs=++-+
  Constant : Constant  Value=-0.0074
  Gain : Gain  Gain=0.00051704
  Gain1 : Gain  Gain=0.0073
  Gain2 : Gain  Gain=0.018
  Multiply : Product
  Square : Math  Operator=square  SaturateOnIntegerOverflow=on
  Ctx : Outport
  wires:
  Add/1 -> Multiply/2
  Gain1/1 -> Add/3
  Miu/1 -> Multiply/1, Gain/1
  Constant/1 -> Add/1
  Gain/1 -> Add/2
  Square/1 -> Gain2/1
  Gain2/1 -> Add/4
  Lumda/1 -> Square/1, Gain1/1
  Multiply/1 -> Ctx/1  "Ctx"

== system test_bu01_2018b_tuning/Plant/bu01_model/动力系统模型/Motor3_TM_P/TM1654P /螺旋桨模型/螺旋桨气动/计算螺旋桨气动系数/计算Cty ==
  Miu : Inport
  Lumda : Inport  Port=2
  Add1 : Sum  Inputs=+++-
  Constant : Constant  Value=3
  Constant1 : Constant  Value=-0.002  OutDataTypeStr=double
  Gain3 : Gain  Gain=0.0103
  Gain4 : Gain  Gain=0.0168
  Gain5 : Gain  Gain=0.0897
  Multiply1 : Product
  Power : Math  Operator=pow  SaturateOnIntegerOverflow=on
  Square2 : Math  Operator=square  SaturateOnIntegerOverflow=on
  Cty : Outport
  wires:
  Gain5/1 -> Add1/4
  Multiply1/1 -> Cty/1  "Cty"
  Gain3/1 -> Add1/2
  Lumda/1 -> Power/1, Square2/1, Gain3/1
  Square2/1 -> Gain4/1
  Constant/1 -> Power/2
  Gain4/1 -> Add1/3
  Add1/1 -> Multiply1/2
  Constant1/1 -> Add1/1
  Power/1 -> Gain5/1
  Miu/1 -> Multiply1/1

== system test_bu01_2018b_tuning/Plant/bu01_model/动力系统模型/Motor3_TM_P/TM1654P /螺旋桨模型/螺旋桨气动/计算螺旋桨气动系数/计算Ctz ==
  Miu : Inport
  Lumda : Inport  Port=2
  Add2 : Sum  Inputs=++-+-
  Add3 : Sum  Inputs=++-+
  Constant3 : Constant  Value=0.0651
  Constant4 : Constant  Value=0.0845
  Gain10 : Gain  Gain=0.0583
  Gain11 : Gain  Gain=0.3529
  Gain6 : Gain  Gain=0.0579
  Gain7 : Gain  Gain=0.0066
  Gain8 : Gain  Gain=-0.2325
  Gain9 : Gain  Gain=0.1346
  Lumda1 : InportShadow  Port=2
  Multiply2 : Product
  Square3 : Math  Operator=square  SaturateOnIntegerOverflow=on
  Square4 : Math  Operator=square  SaturateOnIntegerOverflow=on
  Square5 : Math  Operator=square  SaturateOnIntegerOverflow=on
  Ctz : Outport
  wires:
  Gain7/1 -> Add3/3
  Gain6/1 -> Add3/2
  Multiply2/1 -> Add3/4
  Add3/1 -> Ctz/1  "Ctz"
  Miu/1 -> Square4/1, Gain6/1, Square3/1, Gain8/1
  Lumda/1 -> Square5/1, Gain10/1
  Constant3/1 -> Add3/1
  Add2/1 -> Multiply2/2
  Square4/1 -> Gain9/1
  Constant4/1 -> Add2/3
  Gain9/1 -> Add2/2
  Square5/1 -> Gain11/1
  Gain11/1 -> Add2/5
  Gain8/1 -> Add2/1
  Square3/1 -> Gain7/1
  Gain10/1 -> Add2/4
  Lumda1/1 -> Multiply2/1

== system test_bu01_2018b_tuning/Plant/bu01_model/动力系统模型/Motor4_TM_N/TM1654N /螺旋桨模型/螺旋桨气动/计算螺旋桨气动系数/计算Cmx ==
  Miu : Inport
  Lumda : Inport  Port=2
  Add : Sum  Inputs=++--
  Constant : Constant  Value=0.0101
  Gain : Gain  Gain=0.0041
  Gain1 : Gain  Gain=0.009
  Gain2 : Gain  Gain=0.0032
  Multiply : Product
  Square : Math  Operator=square  SaturateOnIntegerOverflow=on
  Cmx : Outport
  wires:
  Multiply/1 -> Cmx/1  "Cmx"
  Lumda/1 -> Square/1, Gain1/1
  Gain2/1 -> Add/4
  Square/1 -> Gain2/1
  Gain/1 -> Add/2
  Constant/1 -> Add/1
  Miu/1 -> Multiply/1, Gain/1
  Gain1/1 -> Add/3
  Add/1 -> Multiply/2

== system test_bu01_2018b_tuning/Plant/bu01_model/动力系统模型/Motor4_TM_N/TM1654N /螺旋桨模型/螺旋桨气动/计算螺旋桨气动系数/计算Cmy ==
  Miu : Inport
  Lumda : Inport  Port=2
  Add1 : Sum  Inputs=++--
  Constant1 : Constant  Value=0.0101
  Gain1 : Gain  Gain=0.0041
  Gain3 : Gain  Gain=0.009
  Gain4 : Gain  Gain=0.0032
  Multiply1 : Product
  Square2 : Math  Operator=square  SaturateOnIntegerOverflow=on
  Cmy : Outport
  wires:
  Miu/1 -> Multiply1/1, Gain1/1
  Constant1/1 -> Add1/1
  Add1/1 -> Multiply1/2
  Gain4/1 -> Add1/4
  Square2/1 -> Gain4/1
  Lumda/1 -> Square2/1, Gain3/1
  Gain3/1 -> Add1/3
  Multiply1/1 -> Cmy/1  "Cmy"
  Gain1/1 -> Add1/2

== system test_bu01_2018b_tuning/Plant/bu01_model/动力系统模型/Motor4_TM_N/TM1654N /螺旋桨模型/螺旋桨气动/计算螺旋桨气动系数/计算Cmz ==
  Miu : Inport
  Lumda : Inport  Port=2
  Add2 : Sum  Inputs=+-+--
  Add3 : Sum  Inputs=+-++
  Constant3 : Constant  Value=0.0036
  Constant4 : Constant  Value=0.0023
  Gain10 : Gain  Gain=0.0105
  Gain11 : Gain  Gain=0.0078
  Gain6 : Gain  Gain=0.0006554
  Gain7 : Gain  Gain=0.00080732
  Gain8 : Gain  Gain=0.006
  Gain9 : Gain  Gain=0.0043
  Lumda1 : InportShadow  Port=2
  Multiply2 : Product
  Square3 : Math  Operator=square  SaturateOnIntegerOverflow=on
  Square4 : Math  Operator=square  SaturateOnIntegerOverflow=on
  Square5 : Math  Operator=square  SaturateOnIntegerOverflow=on
  Cmz : Outport
  wires:
  Lumda1/1 -> Multiply2/1
  Gain10/1 -> Add2/4
  Square3/1 -> Gain7/1
  Gain8/1 -> Add2/1
  Gain11/1 -> Add2/5
  Square5/1 -> Gain11/1
  Gain9/1 -> Add2/2
  Constant4/1 -> Add2/3
  Square4/1 -> Gain9/1
  Add2/1 -> Multiply2/2
  Constant3/1 -> Add3/1
  Lumda/1 -> Gain10/1, Square5/1
  Miu/1 -> Gain6/1, Square3/1, Square4/1, Gain8/1
  Add3/1 -> Cmz/1  "Cmz"
  Multiply2/1 -> Add3/4
  Gain6/1 -> Add3/2
  Gain7/1 -> Add3/3

== system test_bu01_2018b_tuning/Plant/bu01_model/动力系统模型/Motor4_TM_N/TM1654N /螺旋桨模型/螺旋桨气动/计算螺旋桨气动系数/计算Ctx ==
  Miu : Inport
  Lumda : Inport  Port=2
  Add : Sum  Inputs=++-+
  Constant : Constant  Value=-0.0074
  Gain : Gain  Gain=0.00051704
  Gain1 : Gain  Gain=0.0073
  Gain2 : Gain  Gain=0.018
  Multiply : Product
  Square : Math  Operator=square  SaturateOnIntegerOverflow=on
  Ctx : Outport
  wires:
  Add/1 -> Multiply/2
  Gain1/1 -> Add/3
  Miu/1 -> Multiply/1, Gain/1
  Constant/1 -> Add/1
  Gain/1 -> Add/2
  Square/1 -> Gain2/1
  Gain2/1 -> Add/4
  Lumda/1 -> Square/1, Gain1/1
  Multiply/1 -> Ctx/1  "Ctx"

== system test_bu01_2018b_tuning/Plant/bu01_model/动力系统模型/Motor4_TM_N/TM1654N /螺旋桨模型/螺旋桨气动/计算螺旋桨气动系数/计算Cty ==
  Miu : Inport
  Lumda : Inport  Port=2
  Add1 : Sum  Inputs=+++-
  Constant : Constant  Value=3
  Constant1 : Constant  Value=-0.002  OutDataTypeStr=double
  Gain3 : Gain  Gain=0.0103
  Gain4 : Gain  Gain=0.0168
  Gain5 : Gain  Gain=0.0897
  Multiply1 : Product
  Power : Math  Operator=pow  SaturateOnIntegerOverflow=on
  Square2 : Math  Operator=square  SaturateOnIntegerOverflow=on
  Cty : Outport
  wires:
  Gain5/1 -> Add1/4
  Multiply1/1 -> Cty/1  "Cty"
  Gain3/1 -> Add1/2
  Lumda/1 -> Power/1, Square2/1, Gain3/1
  Square2/1 -> Gain4/1
  Constant/1 -> Power/2
  Gain4/1 -> Add1/3
  Add1/1 -> Multiply1/2
  Constant1/1 -> Add1/1
  Power/1 -> Gain5/1
  Miu/1 -> Multiply1/1

== system test_bu01_2018b_tuning/Plant/bu01_model/动力系统模型/Motor4_TM_N/TM1654N /螺旋桨模型/螺旋桨气动/计算螺旋桨气动系数/计算Ctz ==
  Miu : Inport
  Lumda : Inport  Port=2
  Add2 : Sum  Inputs=++-+-
  Add3 : Sum  Inputs=++-+
  Constant3 : Constant  Value=0.0651
  Constant4 : Constant  Value=0.0845
  Gain10 : Gain  Gain=0.0583
  Gain11 : Gain  Gain=0.3529
  Gain6 : Gain  Gain=0.0579
  Gain7 : Gain  Gain=0.0066
  Gain8 : Gain  Gain=-0.2325
  Gain9 : Gain  Gain=0.1346
  Lumda1 : InportShadow  Port=2
  Multiply2 : Product
  Square3 : Math  Operator=square  SaturateOnIntegerOverflow=on
  Square4 : Math  Operator=square  SaturateOnIntegerOverflow=on
  Square5 : Math  Operator=square  SaturateOnIntegerOverflow=on
  Ctz : Outport
  wires:
  Gain7/1 -> Add3/3
  Gain6/1 -> Add3/2
  Multiply2/1 -> Add3/4
  Add3/1 -> Ctz/1  "Ctz"
  Miu/1 -> Gain8/1, Square4/1, Square3/1, Gain6/1
  Lumda/1 -> Square5/1, Gain10/1
  Constant3/1 -> Add3/1
  Add2/1 -> Multiply2/2
  Square4/1 -> Gain9/1
  Constant4/1 -> Add2/3
  Gain9/1 -> Add2/2
  Square5/1 -> Gain11/1
  Gain11/1 -> Add2/5
  Gain8/1 -> Add2/1
  Square3/1 -> Gain7/1
  Gain10/1 -> Add2/4
  Lumda1/1 -> Multiply2/1
